simulink model "AnalogChannel"  (R2023b)
settings: Solver=VariableStepAuto  StartTime=0.0  StopTime=20  RelTol=1e-3
libraries: dspfdesign x3, dspmathops x2, dspsrcs4 x1

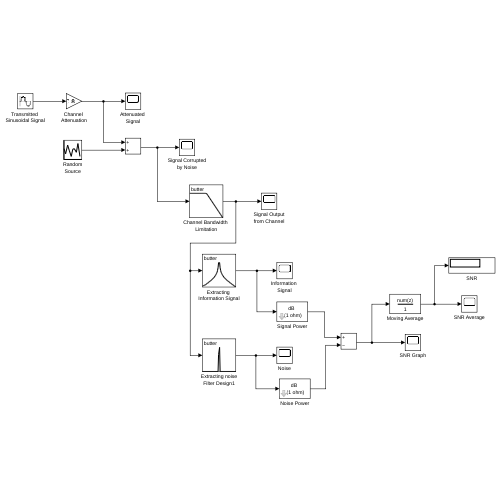
[thumbnail: Simulink's stored preview of the top-level diagram]
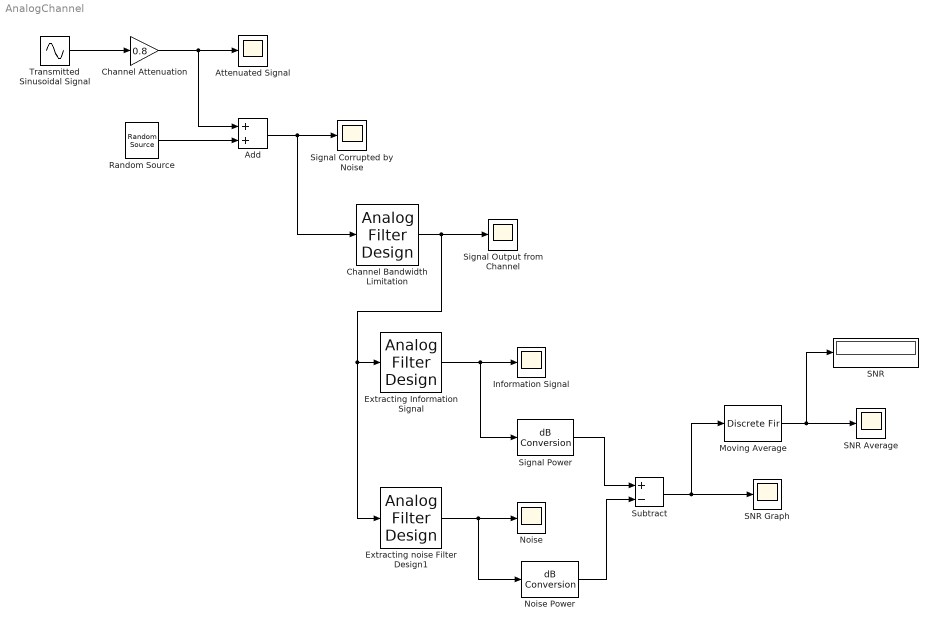
== system AnalogChannel ==
  Add : Sum
  Attenuated Signal : Scope
  Channel Attenuation : Gain  Gain=0.8
  Channel Bandwidth Limitation : dspfdesign/Analog Filter Design  method=Butterworth  filttype=Lowpass  N=10  Wlo=1000  Whi=80  Rp=2  Rs=40
  Extracting Information Signal : dspfdesign/Analog Filter Design  method=Butterworth  filttype=Bandpass  N=10  Wlo=195  Whi=205  Rp=2  Rs=40
  Extracting noise Filter Design1 : dspfdesign/Analog Filter Design  method=Butterworth  filttype=Bandstop  N=10  Wlo=195  Whi=205  Rp=2  Rs=40
  Information Signal : Scope
  Moving Average : DiscreteFir  Coefficients=ones(1,1000)/1000
  Noise : Scope
  Noise Power : dspmathops/dB Conversion  dBtype=dB  intype=Amplitude  R=1  fuzz=off
  Random Source : dspsrcs4/Random Source  SrcType=Gaussian  NormMethod=Ziggurat  CltLength=12  MinVal=0  MaxVal=1  MeanVal=0  VarVal=1  RepMode=Not repeatable  rawSeed=1  IsInherit=off  SampMode=Discrete  SampTime=0.001  SampFrame=1  DataType=Double  OutComplex=Real  OutputFrames=off
  SNR : Display
  SNR Average : Scope
  SNR Graph : Scope
  Signal Corrupted by Noise : Scope
  Signal Output from Channel : Scope
  Signal Power : dspmathops/dB Conversion  dBtype=dB  intype=Amplitude  R=1  fuzz=off
  Subtract : Sum  Inputs=+-
  Transmitted Sinusoidal Signal : Sin  Amplitude=10  Frequency=200  SampleTime=0.001
  wires:
  Transmitted Sinusoidal Signal/1 -> Channel Attenuation/1
  Channel Attenuation/1 -> Attenuated Signal/1, Add/1
  Random Source/1 -> Add/2
  Add/1 -> Signal Corrupted by Noise/1, Channel Bandwidth Limitation/1
  Channel Bandwidth Limitation/1 -> Extracting noise Filter Design1/1, Extracting Information Signal/1, Signal Output from Channel/1
  Extracting Information Signal/1 -> Signal Power/1, Information Signal/1
  Extracting noise Filter Design1/1 -> Noise/1, Noise Power/1
  Noise Power/1 -> Subtract/2
  Signal Power/1 -> Subtract/1
  Subtract/1 -> SNR Graph/1, Moving Average/1
  Moving Average/1 -> SNR Average/1, SNR/1
